simulink model "respeldoRXBLE"  (R2020a)
settings: Solver=VariableStepAuto  StartTime=0.0  StopTime=10.0  RelTol=1e-3
undefined symbols (not defined in the file): BLE_Receive, BLE_Send, blue, blue2, blue3, Contador, dato_2, green, green2, green3, intentRecBle, red, red2, red3, reset, Size_received
libraries: simulink x4, androiduilib x4, androidaudiovideolib x3, androidcommunicationlib x2, dspswit3 x1
settings Model: Creator=luisi  LastModifiedBy=luisi

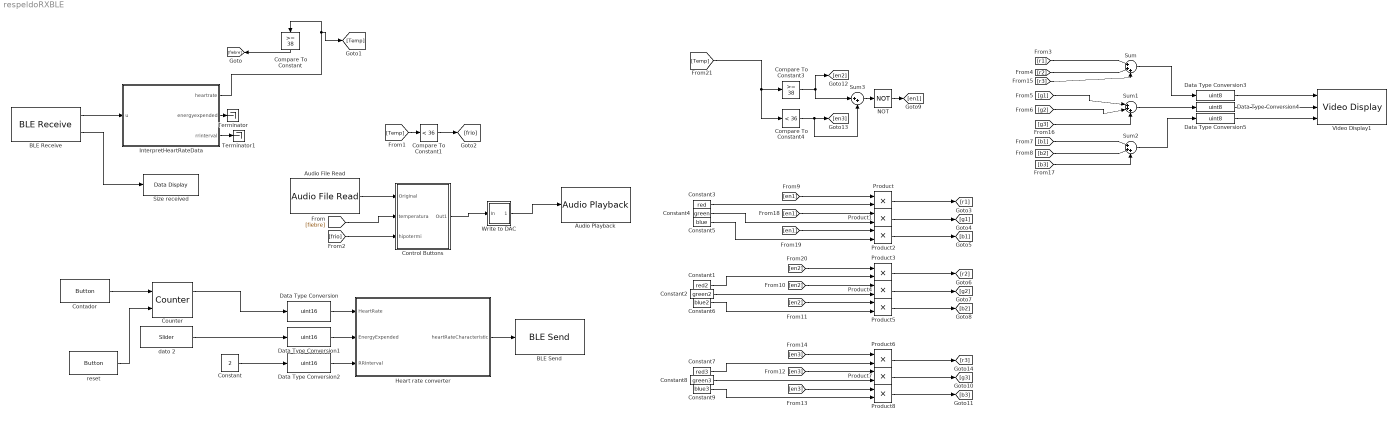
== system respeldoRXBLE ==
  Audio File Read : androidaudiovideolib/Audio File Read  FileName=C:\Users\luisi\Downloads\baby.mp3  FrameSize=4410
      settings: SourceProductBaseCode=ANDROID
  Audio Playback : androidaudiovideolib/Audio Playback  SampleFreq=44100  AudioSamplingFreq=44100  SampleTime=0.1  DeviceStr=0  QueueDuration=0  BlockPlatform=Android
      settings: SourceProductBaseCode=ANDROID
  BLE Receive : androidcommunicationlib/BLE Receive  DeviceMode=Central (Client)  BluetoothAddress=43:33:83:91:21:94  CharUUID=00002a37-0000-1000-8000-00805f9b34fb  ServiceUUID=0000180d-0000-1000-8000-00805f9b34fb  device=RedmiLuisa  character="Heart Rate\\Heart Rate  Measurement"  CustomService=off  ServiceName=Heart Rate  CharacteristicName="Heart Rate  Measurement"  CustomServiceUUID=<Enter Service UUID>  CustomCharUUID=<Enter Characteristic UUID>  DataSize=7  SampleTime=0.1  charseruuid=00001801-0000-1000-8000-00805f9b34fb\00002a05-0000-1000-8000-00805f9b34fb  seruuid=00001810-0000-1000-8000-00805f9b34fb  PeripheralService=0000180d-0000-1000-8000-00805f9b34fb  PeripheralCharacteristic=00002a37-0000-1000-8000-00805f9b34fb  chruuid=00002a37-0000-1000-8000-00805f9b34fb  BLEId=intentRecBle/BLE_Receive  Devicename=RedmiLuisa  IsCustomService=0
      settings: SourceProductBaseCode=ANDROID
  BLE Send : androidcommunicationlib/BLE Send  DeviceMode=Peripheral (Server)  BluetoothAddress=43:33:83:91:21:94  CharUUID=00002a05-0000-1000-8000-00805f9b34fb  ServiceUUID=00001801-0000-1000-8000-00805f9b34fb  device=RedmiLuisa  character=Generic Attribute\Service Changed  CustomService=off  ServiceName=Heart Rate  CharacteristicName="Heart Rate  Measurement"  CustomServiceUUID=<Enter Service UUID>  CustomCharUUID=<Enter Characteristic UUID>  charseruuid=00001801-0000-1000-8000-00805f9b34fb\00002a05-0000-1000-8000-00805f9b34fb  seruuid=00001810-0000-1000-8000-00805f9b34fb  chruuid=00002a37-0000-1000-8000-00805f9b34fb  PeripheralService=0000180d-0000-1000-8000-00805f9b34fb  PeripheralCharacteristic=00002a37-0000-1000-8000-00805f9b34fb  BLEId=intentRecBle/BLE_Send  Devicename=RedmiLuisa  IsCustomService=0  Size=-1
      settings: SourceProductBaseCode=ANDROID
  Compare To Constant : simulink/Logic and Bit Operations/Compare To Constant  relop=>=  const=38  OutDataTypeStr=boolean
  Compare To Constant1 : simulink/Logic and Bit Operations/Compare To Constant  relop=<  const=36  OutDataTypeStr=boolean
  Compare To Constant3 : simulink/Logic and Bit Operations/Compare To Constant  relop=>=  const=38  OutDataTypeStr=uint8
  Compare To Constant4 : simulink/Logic and Bit Operations/Compare To Constant  relop=<  const=36  OutDataTypeStr=uint8
  Constant : Constant  Value=2
  Constant1 : Constant  Value=red2
  Constant2 : Constant  Value=green2
  Constant3 : Constant  Value=red
  Constant4 : Constant  Value=green
  Constant5 : Constant  Value=blue
  Constant6 : Constant  Value=blue2
  Constant7 : Constant  Value=red3
  Constant8 : Constant  Value=green3
  Constant9 : Constant  Value=blue3
  Contador : androiduilib/Button  ButtonState=Not pressed  ButtonId=intentRecBle/Contador  State=off  SampleTime=0.1  BlockPlatform=Android
      settings: SourceProductBaseCode=ANDROID
  Control Buttons : Subsystem
  Counter : dspswit3/Counter  Direction=Up  CountEvent=Rising edge  CounterSize=User defined  MaxCount=255  InitialCount=0  Output=Count and Hit  HitValue=32  ResetInput=on  SamplesPerFrame=1  Ts=1  CntDtype=double  HitDtype=Logical
  Data Type Conversion : DataTypeConversion  OutDataTypeStr=uint16
  Data Type Conversion1 : DataTypeConversion  OutDataTypeStr=uint16
  Data Type Conversion2 : DataTypeConversion  OutDataTypeStr=uint16
  Data Type Conversion3 : DataTypeConversion  OutDataTypeStr=uint8
  Data Type Conversion4 : DataTypeConversion  OutDataTypeStr=uint8
  Data Type Conversion5 : DataTypeConversion  OutDataTypeStr=uint8
  Heart rate converter : MATLAB Function  TreatAsAtomicUnit=on
  InterpretHeartRateData : MATLAB Function  TreatAsAtomicUnit=on
  NOT : Logic  Operator=NOT  IconShape=distinctive  AllPortsSameDT=off  OutDataTypeStr=boolean
  Product{,1..8} (9 alike) : Product
  Size received : androiduilib/Data Display  DataDisplayId=intentRecBle/Size_received  Format=Float  Precision=6  SimulateUsing=Code generation  blockPlatform=Android
      settings: SourceProductBaseCode=ANDROID
  Sum : Sum  Inputs=|+++
  Sum1 : Sum  Inputs=|+++
  Sum2 : Sum  Inputs=|+++
  Sum3 : Sum  Inputs=|++
  Terminator : Terminator
  Terminator1 : Terminator
  Video Display1 : androidaudiovideolib/Video Display  BlockPlatform=Android
      settings: SourceProductBaseCode=ANDROID
  Write to DAC : Subsystem
  dato 2 : androiduilib/Slider  Min=0  Value=0  Max=5  Resolution=1  SliderId=intentRecBle/dato_2  SampleTime=0.1  BlockPlatform=Android
      settings: SourceProductBaseCode=ANDROID
  reset : androiduilib/Button  ButtonState=Not pressed  ButtonId=intentRecBle/reset  State=off  SampleTime=0.1  BlockPlatform=Android
      settings: SourceProductBaseCode=ANDROID
  wires:
  Constant7/1 -> Product6/2
  Data Type Conversion2/1 -> Heart rate converter/3(RRInterval)
  [Temp] -> Compare To Constant1/1
  Compare To Constant/1 -> [fiebre]
  Constant1/1 -> Product3/2
  Constant/1 -> Data Type Conversion2/1
  BLE Receive/1 -> InterpretHeartRateData/1(u)
  Heart rate converter/1(heartRateCharacteristic) -> BLE Send/1
  InterpretHeartRateData/3(rrinterval) -> Terminator1/1
  Audio File Read/1 -> Control Buttons/1(Original)
  BLE Receive/2 -> Size received/1
  [b3] -> Sum2/3
  reset/1 -> Counter/2
  Constant5/1 -> Product2/2
  Product4/1 -> [g2]
  Sum3/1 -> NOT/1
  [en1] -> Product1/1
  Sum1/1 -> Data Type Conversion4/1
  Product8/1 -> [b3]
  Constant8/1 -> Product7/2
  Contador/1 -> Counter/1
  Constant2/1 -> Product4/2
  Data Type Conversion4/1 -> Video Display1/2
  [b1] -> Sum2/1
  Counter/1 -> Data Type Conversion/1
  Constant4/1 -> Product1/2
  Product5/1 -> [b2]
  [r1] -> Sum/1
  [g1] -> Sum1/1
  Product2/1 -> [b1]
  Write to DAC/1(Out) -> Audio Playback/1
  Sum/1 -> Data Type Conversion3/1
  Constant6/1 -> Product5/2
  [en3] -> Product8/1
  [en1] -> Product/1
  InterpretHeartRateData/1(heartrate) -> [Temp], Compare To Constant/1
  dato 2/1 -> Data Type Conversion1/1
  Compare To Constant1/1 -> [frio]
  Product3/1 -> [r2]
  [fiebre] -> Control Buttons/2(temperatura)
  Constant3/1 -> Product/2
  [r2] -> Sum/2
  Product/1 -> [r1]
  [en3] -> Product6/1
  [b2] -> Sum2/2
  Compare To Constant3/1 -> Sum3/1, [en2]
  [en2] -> Product5/1
  [en1] -> Product2/1
  Constant9/1 -> Product8/2
  Data Type Conversion1/1 -> Heart rate converter/2(EnergyExpended)
  [en2] -> Product4/1
  NOT/1 -> [en1]
  [r3] -> Sum/3
  Data Type Conversion3/1 -> Video Display1/1
  Product6/1 -> [r3]
  [en3] -> Product7/1
  Data Type Conversion5/1 -> Video Display1/3
  Data Type Conversion/1 -> Heart rate converter/1(HeartRate)
  InterpretHeartRateData/2(energyexpended) -> Terminator/1
  [g2] -> Sum1/2
  Sum2/1 -> Data Type Conversion5/1
  Product7/1 -> [g3]
  [Temp] -> Compare To Constant4/1, Compare To Constant3/1
  [frio] -> Control Buttons/3(hipotermi)
  [en2] -> Product3/1
  Product1/1 -> [g1]
  Compare To Constant4/1 -> [en3], Sum3/2
  Control Buttons/1(Out1) -> Write to DAC/1(In)
  [g3] -> Sum1/3

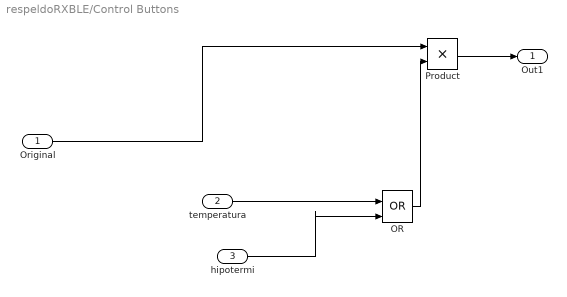
== system respeldoRXBLE/Control Buttons ==
  Original : Inport
  temperatura : Inport  Port=2
  hipotermi : Inport  Port=3
  OR : Logic  Operator=OR  IconShape=distinctive  AllPortsSameDT=off  OutDataTypeStr=boolean
  Product : Product
  Out1 : Outport  VectorParamsAs1DForOutWhenUnconnected=off
  wires:
  Product/1 -> Out1/1
  Original/1 -> Product/1
  temperatura/1 -> OR/1
  hipotermi/1 -> OR/2
  OR/1 -> Product/2

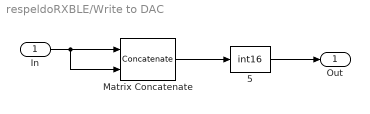
== system respeldoRXBLE/Write to DAC ==
  In : Inport
  " 5" : DataTypeConversion  OutDataTypeStr=int16
  Matrix Concatenate : Concatenate  Mode=Multidimensional array  ConcatenateDimension=2
  Out : Outport  VectorParamsAs1DForOutWhenUnconnected=off
  wires:
  In/1 -> Matrix Concatenate/2, Matrix Concatenate/1
  Matrix Concatenate/1 -> " 5"/1
  " 5"/1 -> Out/1

== matlab function respeldoRXBLE/Heart rate converter ==
  data: HeartRate input; heartRateCharacteristic output; EnergyExpended input; RRInterval input
function heartRateCharacteristic = ConvertToHeartRateFormat(HeartRate, EnergyExpended, RRInterval)
flag = uint8(25);
heartRateCharacteristic = zeros(7,1,'uint8');
heartRateCharacteristic(1)= flag;
[lower, upper] = getBytes(HeartRate);
heartRateCharacteristic(2) = lower;
heartRateCharacteristic(3) = upper;
[lower, upper] = getBytes(EnergyExpended);
heartRateCharacteristic(4) = lower;
heartRateCharacteristic(5) = upper;
[lower, upper] = getBytes(RRInterval);
heartRateCharacteristic(6) = lower;
heartRateCharacteristic(7) = upper;
end

function [lower,upper] = getBytes(parameter)
h = dec2bin(parameter,16);
lower = bin2dec(h(9:16));
upper= bin2dec(h(1:8));
end

== matlab function respeldoRXBLE/InterpretHeartRateData ==
  data: u input; heartrate output; energyexpended output; rrinterval output
function [heartrate, energyexpended, rrinterval ] = InterpretHeartRateData(u)
flag = uint8(u(1));
heartrate = uint16(0);
energyexpended=uint16(0);
rrinterval = uint16(0);
b = bitget(flag,8:-1:1);

 if b(8) == 0
     format = uint8(2);
     heartrate = uint16(u(2));
 else
     format = uint8(3);
     heartrate = typecast([u(2) u(3)], 'uint16');
 end
 
 if b(5) == 1
     energy = uint8(2);
     energyexpended = typecast([u(format +1) u(format + 2)], 'uint16');
 else
     energy = uint8(0);
     energyexpended = uint16(0);
 end
 
 if b(4) == 1
     rrinterval = typecast([u(format +energy + 1) u(format + energy + 2)],'uint16');
 else
     rrinterval = uint16(0);
 end
end
